simulink model "ev_phase2"  (R2025a)
settings: Solver=VariableStepAuto  StartTime=0.0  StopTime=3600  RelTol=1e-3
libraries: SignalEditorBlockLib x1
settings Model: Creator=piyus  LastModifiedBy=piyus

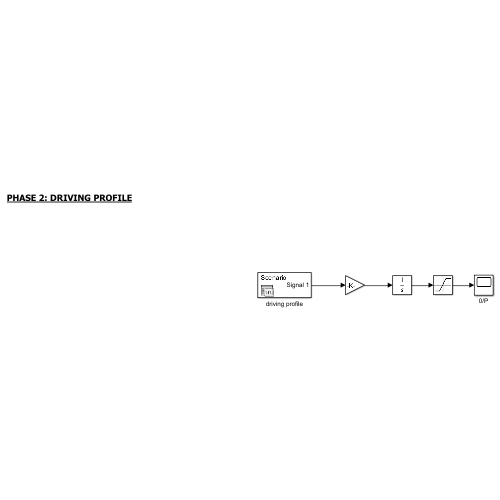
[thumbnail: Simulink's stored preview of the top-level diagram]
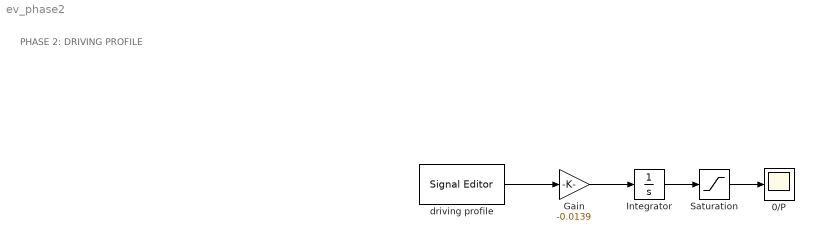
== system ev_phase2 ==
  note: PHASE 2: DRIVING PROFILE
  0/P : Scope
      settings: ActiveDisplayYMinimum=-124.65492788290996  ActiveDisplayYMaximum=150.97007211708981
  Gain : Gain  Gain=-0.0139
  Integrator : Integrator  InitialCondition=100
  Saturation : Saturate  UpperLimit=100  LowerLimit=0
  driving profile : SignalEditorBlockLib/Signal Editor  FileName=driving_profile.mat  ActiveScenario=Scenario  ActiveSignal=Signal 1  IsBus=off  OutputBusObjectStr=Bus: BusObject  SampleTime=0  ZeroCross=off  OutputAfterFinalValue=Setting to zero  Unit=inherit  PreserveSignalName=on  ApplySigPropsToAllScenarios=on  ApplySigPropsToAllSignals=off  SignalPropertySource=Dialog parameters
  wires:
  Saturation/1 -> 0/P/1
  Gain/1 -> Integrator/1
  Integrator/1 -> Saturation/1
  driving profile/1 -> Gain/1
